simulink library "MyLibTwoSwitchConfig"  (R2024a)
settings: Solver=VariableStepAuto  StartTime=0.0  StopTime=10.0  RelTol=1e-3
values from neighbouring files (symbols this model uses):
  cnt_min = 10    [TX_PM_MODEL_Setup.m]
  cnt_n_bits = 9    [TX_PM_MODEL_Setup.m]
  fH = 2*pi * (fin) / (2*pi - pi/2/N_PHASE_CYCLES)    (= 1066666.66667)    [TX_PM_MODEL_Setup.m]
  fin = 1e6    (= 1000000)    [TX_PM_MODEL_Setup.m]
  fL = 2*pi * (fin) / (2*pi + pi/2/N_PHASE_CYCLES)    (= 941176.470588)    [TX_PM_MODEL_Setup.m]
  R = 0.2    [TX_PM_MODEL_Setup.m]
  tcmp = 5    [TX_PM_MODEL_Setup.m]
  VDD = 5    [Oscillator_Setup.m]    (also in TX_PM_MODEL_Setup.m = 10)
libraries: fl_lib x26, nesl_utility x16, ee_lib x2
settings Model: Creator=ciano  LastModifiedBy=ciano

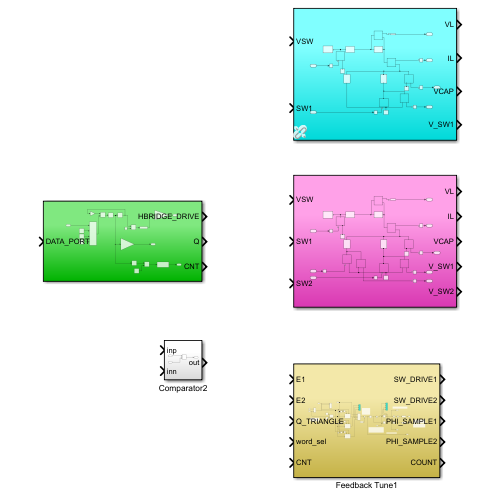
[thumbnail: Simulink's stored preview of the top-level diagram]
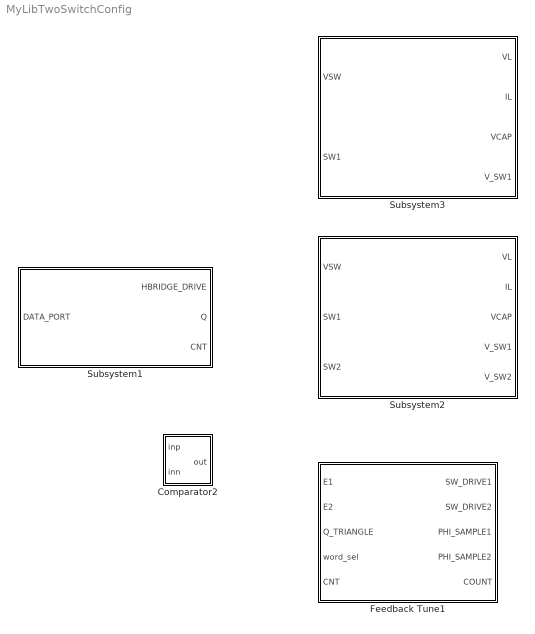
== system MyLibTwoSwitchConfig ==
  Comparator2 : Subsystem
  Feedback Tune1 : Subsystem
  Subsystem1 : Subsystem
  Subsystem2 : Subsystem
  Subsystem3 : Subsystem  AncestorBlock=MyLibTwoSwitchConfig/Subsystem2

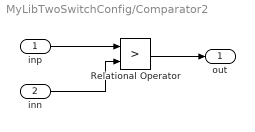
== system MyLibTwoSwitchConfig/Comparator2 ==
  inp : Inport
  inn : Inport  Port=2
  Relational Operator : RelationalOperator  Operator=>  OutDataTypeStr=boolean  RndMeth=Simplest  InputSameDT=off
  out : Outport
  wires:
  inp/1 -> Relational Operator/1
  Relational Operator/1 -> out/1
  inn/1 -> Relational Operator/2

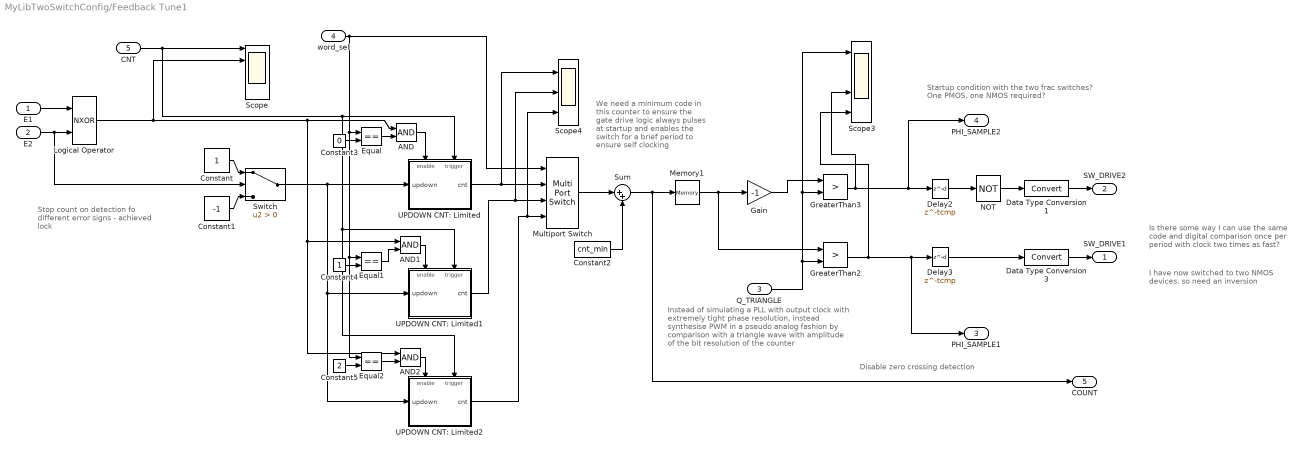
== system MyLibTwoSwitchConfig/Feedback Tune1 ==
  note: Is there some way I can use the same code and digital comparison once per period with clock two times as fast?
  note: We need a minimum code in this counter to ensure the gate drive logic always pulses at startup and enables the switch for a brief period to ensure self clocking
  note: Disable zero crossing detection
  note: Instead of simulating a PLL with output clock with extremely tight phase resolution, instead synthesise PWM in a pseudo analog fashion by comparison with a triangle wave with amplitude of the bit resolution of the counter
  note: Stop count on detection fo different error signs - achieved lock
  note: Startup condition with the two frac switches?
      | One PMOS, one NMOS required?
  note: I have now switched to two NMOS devices. so need an inversion
  E1 : Inport
  E2 : Inport  Port=2
  Q_TRIANGLE : Inport  Port=3
  word_sel : Inport  Port=4
  CNT : Inport  Port=5
  AND : Logic  IconShape=distinctive  AllPortsSameDT=off  OutDataTypeStr=boolean
  AND1 : Logic  IconShape=distinctive  AllPortsSameDT=off  OutDataTypeStr=boolean
  AND2 : Logic  IconShape=distinctive  AllPortsSameDT=off  OutDataTypeStr=boolean
  Constant : Constant
  Constant1 : Constant  Value=-1
  Constant2 : Constant  Value=cnt_min
  Constant3 : Constant  Value=0
  Constant4 : Constant
  Constant5 : Constant  Value=2
  Data Type Conversion1 : DataTypeConversion  SaturateOnIntegerOverflow=off  RndMeth=Floor
  Data Type Conversion3 : DataTypeConversion  SaturateOnIntegerOverflow=off  RndMeth=Floor
  Delay2 : Delay  DelayLength=tcmp  SampleTime=1e-9
  Delay3 : Delay  DelayLength=tcmp  SampleTime=1e-9
  Equal : RelationalOperator  Operator===  OutDataTypeStr=boolean  RndMeth=Simplest  InputSameDT=off
  Equal1 : RelationalOperator  Operator===  OutDataTypeStr=boolean  RndMeth=Simplest  InputSameDT=off
  Equal2 : RelationalOperator  Operator===  OutDataTypeStr=boolean  RndMeth=Simplest  InputSameDT=off
  Gain : Gain  Gain=-1
  GreaterThan2 : RelationalOperator  Operator=>  OutDataTypeStr=boolean  ZeroCross=off  RndMeth=Simplest  InputSameDT=off
  GreaterThan3 : RelationalOperator  Operator=>  OutDataTypeStr=boolean  ZeroCross=off  RndMeth=Simplest  InputSameDT=off
  Logical Operator : Logic  Operator=NXOR  AllPortsSameDT=off  OutDataTypeStr=boolean
  Memory1 : Memory
  Multiport Switch : MultiPortSwitch  DataPortOrder=Zero-based contiguous  zeroidx=on  SaturateOnIntegerOverflow=off  InputSameDT=off
  NOT : Logic  Operator=NOT  IconShape=distinctive  AllPortsSameDT=off  OutDataTypeStr=boolean
  Scope : Scope  NumInputPorts=5
  Scope3 : Scope  NumInputPorts=4
  Scope4 : Scope  NumInputPorts=3
  Sum : Sum  Inputs=|++
  Switch : Switch  Criteria=u2 > Threshold  ZeroCross=off  SaturateOnIntegerOverflow=off  InputSameDT=off
  UPDOWN CNT: Limited : Subsystem
  UPDOWN CNT: Limited1 : Subsystem
  UPDOWN CNT: Limited2 : Subsystem
  SW_DRIVE1 : Outport
  SW_DRIVE2 : Outport  Port=2
  PHI_SAMPLE1 : Outport  Port=3
  PHI_SAMPLE2 : Outport  Port=4
  COUNT : Outport  Port=5
  wires:
  NOT/1 -> Data Type Conversion1/1
  Gain/1 -> GreaterThan3/1
  GreaterThan3/1 -> Scope3/3, Delay2/1, PHI_SAMPLE2/1
  Delay2/1 -> NOT/1
  E1/1 -> Logical Operator/1
  Equal2/1 -> AND2/2
  AND2/1 -> UPDOWN CNT: Limited2/Enable
  Equal1/1 -> AND1/2
  AND1/1 -> UPDOWN CNT: Limited1/Enable
  Equal/1 -> AND/2
  AND/1 -> UPDOWN CNT: Limited/Enable
  Logical Operator/1 -> Scope/2, AND1/1, AND2/1, AND/1
  E2/1 -> Logical Operator/2, Switch/2
  Constant5/1 -> Equal2/2
  Constant4/1 -> Equal1/2
  Constant3/1 -> Equal/2
  UPDOWN CNT: Limited2/1(cnt) -> Multiport Switch/4, Scope4/3
  UPDOWN CNT: Limited1/1(cnt) -> Multiport Switch/3, Scope4/2
  CNT/1 -> Scope/1, UPDOWN CNT: Limited1/Trigger, UPDOWN CNT: Limited2/Trigger, UPDOWN CNT: Limited/Trigger
  Sum/1 -> Memory1/1, COUNT/1
  Multiport Switch/1 -> Sum/1
  Constant2/1 -> Sum/2
  word_sel/1 -> Multiport Switch/1, Equal/1, Equal1/1, Equal2/1
  Q_TRIANGLE/1 -> GreaterThan2/2, Scope3/1, GreaterThan3/2
  GreaterThan2/1 -> Scope3/4, Delay3/1, PHI_SAMPLE1/1
  Delay3/1 -> Data Type Conversion3/1
  Data Type Conversion1/1 -> SW_DRIVE2/1
  Data Type Conversion3/1 -> SW_DRIVE1/1
  Constant1/1 -> Switch/3
  Constant/1 -> Switch/1
  Switch/1 -> UPDOWN CNT: Limited1/1(updown), UPDOWN CNT: Limited2/1(updown), UPDOWN CNT: Limited/1(updown)
  UPDOWN CNT: Limited/1(cnt) -> Multiport Switch/2, Scope4/1
  Memory1/1 -> GreaterThan2/1, Gain/1

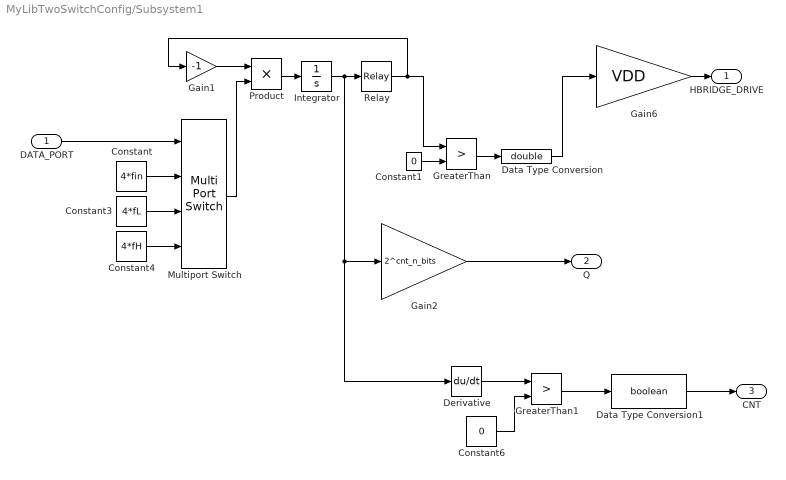
== system MyLibTwoSwitchConfig/Subsystem1 ==
  DATA_PORT : Inport
  Constant : Constant  Value=4*fin
  Constant1 : Constant  Value=0
  Constant3 : Constant  Value=4*fL
  Constant4 : Constant  Value=4*fH
  Constant6 : Constant  Value=0
  Data Type Conversion : DataTypeConversion  OutDataTypeStr=double  SaturateOnIntegerOverflow=off  RndMeth=Floor
  Data Type Conversion1 : DataTypeConversion  OutDataTypeStr=boolean  SaturateOnIntegerOverflow=off  RndMeth=Floor
  Derivative : Derivative
  Gain1 : Gain  Gain=-1
  Gain2 : Gain  Gain=2^cnt_n_bits
  Gain6 : Gain  Gain=VDD
  GreaterThan : RelationalOperator  Operator=>  OutDataTypeStr=boolean  RndMeth=Simplest  InputSameDT=off
  GreaterThan1 : RelationalOperator  Operator=>  OutDataTypeStr=boolean  ZeroCross=off  RndMeth=Simplest  InputSameDT=off
  Integrator : Integrator
  Multiport Switch : MultiPortSwitch  DataPortOrder=Zero-based contiguous  zeroidx=on  SaturateOnIntegerOverflow=off  InputSameDT=off
  Product : Product
  Relay : Relay  OnSwitchValue=1  OffSwitchValue=-1  OffOutputValue=-1
  HBRIDGE_DRIVE : Outport
  Q : Outport  Port=2
  CNT : Outport  Port=3
  wires:
  Gain6/1 -> HBRIDGE_DRIVE/1
  Constant1/1 -> GreaterThan/2
  GreaterThan/1 -> Data Type Conversion/1
  Data Type Conversion/1 -> Gain6/1
  Relay/1 -> Gain1/1, GreaterThan/1
  DATA_PORT/1 -> Multiport Switch/1
  Gain2/1 -> Q/1
  Product/1 -> Integrator/1
  Constant3/1 -> Multiport Switch/3
  Integrator/1 -> Relay/1, Derivative/1, Gain2/1
  Constant4/1 -> Multiport Switch/4
  Constant/1 -> Multiport Switch/2
  Multiport Switch/1 -> Product/2
  Gain1/1 -> Product/1
  Data Type Conversion1/1 -> CNT/1
  Constant6/1 -> GreaterThan1/2
  Derivative/1 -> GreaterThan1/1
  GreaterThan1/1 -> Data Type Conversion1/1

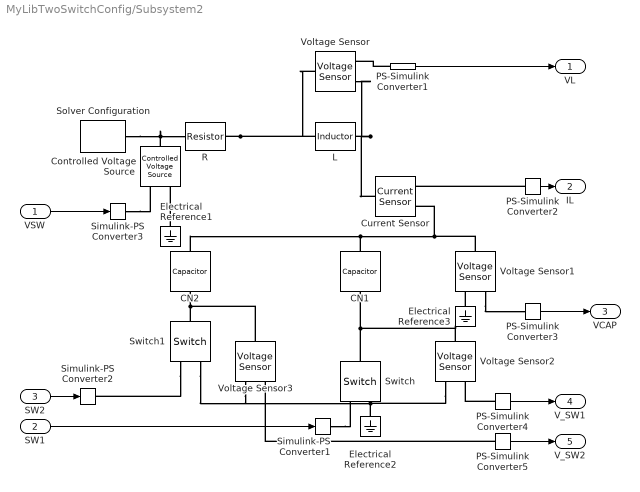
== system MyLibTwoSwitchConfig/Subsystem2 ==
  VSW : Inport
  SW1 : Inport  Port=2
  SW2 : Inport  Port=3
  CN1 : fl_lib/Electrical/Electrical Elements/Capacitor  c=3e-9 F  r=1e-6 Ohm  g=0 1/Ohm  i_specify=off  i_priority=None  i=0 A  i_nominal_specify=off  i_nominal_value=1  i_nominal_unit=A  v_specify=off  v_priority=None  v=0 V  v_nominal_specify=off  v_nominal_value=1  v_nominal_unit=V  vc_specify=off  vc_priority=High  vc=0 V  vc_nominal_specify=off  vc_nominal_value=1  vc_nominal_unit=V
  CN2 : fl_lib/Electrical/Electrical Elements/Capacitor  c=3e-9 F  r=1e-6 Ohm  g=0 1/Ohm  i_specify=off  i_priority=None  i=0 A  i_nominal_specify=off  i_nominal_value=1  i_nominal_unit=A  v_specify=off  v_priority=None  v=0 V  v_nominal_specify=off  v_nominal_value=1  v_nominal_unit=V  vc_specify=off  vc_priority=High  vc=0 V  vc_nominal_specify=off  vc_nominal_value=1  vc_nominal_unit=V
  Controlled Voltage Source : fl_lib/Electrical/Electrical Sources/Controlled Voltage Source
  Current Sensor : fl_lib/Electrical/Electrical Sensors/Current Sensor
  Electrical Reference1 : fl_lib/Electrical/Electrical Elements/Electrical Reference
  Electrical Reference2 : fl_lib/Electrical/Electrical Elements/Electrical Reference
  Electrical Reference3 : fl_lib/Electrical/Electrical Elements/Electrical Reference
  L : ee_lib/Passive/Inductor  l=L H  enable_L_tol=ee.enum.toleranceApplication.none  L_tol=20  tol_distribution=ee.enum.toleranceDistribution.uniform  nSigma=4  r=0 Ohm  g=1e-9 1/Ohm  enable_operating_limits=ee.enum.enable.no  operating_limit_action=ee.enum.passive.reportOpLim.warn  max_working_current=1 A  power_rating=1 W  enable_faults=ee.enum.enable.no  fault_action=simscape.enum.assert.action.none  lambdaPercent=50  k_faulted=0.9999  turnsShort=ee.enum.passive.inductor.turnsShortOption.no  openCct=ee.enum.enable.no  groundShort=ee.enum.passive.inductor.groundShortOption.no  groundShortG=0 1/Ohm  tau_fault=1e-3 s  fault_trigger=ee.enum.faults.faultTrigger.temporal  t_fault=1 s  max_permissible_voltage=100 V  n_fail_on_voltage=1  max_permissible_current=1 A  t_fail_on_current=1 s  i_L_specify=off  i_L_priority=High  i_L=0 A  i_L_nominal_specify=off  i_L_nominal_value=1  i_L_nominal_unit=A  faulted_specify=off  faulted_priority=None  faulted=0
  PS-Simulink Converter{1..5} (5 alike) : nesl_utility/PS-Simulink Converter  PhysicalDomain=network_engine_domain  SubClassName=ps_output  LeftPortType=input  RightPortType=output  PseudoPeriodic=off  Frequencies=[]  VectorFormat=inherit  Unit=inherit  AffineConversion=off
  R : fl_lib/Electrical/Electrical Elements/Resistor  R=R Ohm  i_specify=off  i_priority=None  i=0 A  i_nominal_specify=off  i_nominal_value=1  i_nominal_unit=A  v_specify=off  v_priority=None  v=0 V  v_nominal_specify=off  v_nominal_value=1  v_nominal_unit=V
  Simulink-PS Converter1 : nesl_utility/Simulink-PS Converter  PhysicalDomain=network_engine_domain  SubClassName=ps_input  LeftPortType=input  RightPortType=output  PseudoPeriodic=off  Frequencies=[]  NoiseDistribution=none  NoiseParameters=[]  Unit=1  AffineConversion=off  FilteringAndDerivatives=provide  SimscapeFilterOrder=1  InputFilterTimeConstant=0.001  UdotUserProvided=0
  Simulink-PS Converter2 : nesl_utility/Simulink-PS Converter  PhysicalDomain=network_engine_domain  SubClassName=ps_input  LeftPortType=input  RightPortType=output  PseudoPeriodic=off  Frequencies=[]  NoiseDistribution=none  NoiseParameters=[]  Unit=1  AffineConversion=off  FilteringAndDerivatives=provide  SimscapeFilterOrder=1  InputFilterTimeConstant=0.001  UdotUserProvided=0
  Simulink-PS Converter3 : nesl_utility/Simulink-PS Converter  PhysicalDomain=network_engine_domain  SubClassName=ps_input  LeftPortType=input  RightPortType=output  PseudoPeriodic=off  Frequencies=[]  NoiseDistribution=none  NoiseParameters=[]  Unit=1  AffineConversion=off  FilteringAndDerivatives=provide  SimscapeFilterOrder=1  InputFilterTimeConstant=0.001  UdotUserProvided=0
  Solver Configuration : nesl_utility/Solver Configuration  PhysicalDomain=network_engine_domain  SubClassName=solver  LeftPortType=input  RightPortType=generic  Tones=[]  Harmonics=[]  SimulateNoise=off  Profile=off  UseLocalSampling=off  EnableSwitchedLinearOptims=on  FrequencyDomain=off  UseCCode=off  RelTol=0.001  AbsTol=0.001  MinStep=1e-09  ToWorkspace=off  RevertToSquareIcSolve=off  NumHomotopyIterations=100  PhasorMode=off  PhasorModeNumHarmonics=1  ConsistencySolver=NEWTON_XTOL_AFTER_FTOL  IndexReductionMethod=DerivativeReplacement  DoDC=off  ResidualTolerance=1e-09  ConsistencyTolSource=GLOBAL  ConsistencyAbsTol=0.001  ConsistencyRelTol=0.001  ConsistencyTolFactor=0.001  UseLocalSolver=off  LocalSolverChoice=NE_BACKWARD_EULER_ADVANCER  ResolveIndetEquations=on  FunctionEvalNumThread=1  LocalSolverSampleTime=0.001  DoFixedCost=off  MaxNonlinIter=3  MaxModeIter=2  ComputeImpulses=off  ImpulseIterations=2  LinearAlgebra=auto  LinearAlgebraNumThread=0  EquationFormulation=NE_TIME_EF  DelaysMemoryBudget=1024  AutomaticFiltering=on  FilteringTimeConstant=0.001  PartitionStorageMethod=AS_NEEDED  PartitionMemoryBudget=1024  PartitionMethod=ROBUST  MultibodyUseLocalSolver=off  MultibodyLocalSolverChoice=ODE1  MultibodyLocalSolverSampleTime=0.001
  Switch : fl_lib/Electrical/Electrical Elements/Switch  R_closed=0.1 Ohm  G_open=1e-8 1/Ohm  Threshold=0.5  i_specify=off  i_priority=None  i=0 A  i_nominal_specify=off  i_nominal_value=1  i_nominal_unit=A  v_specify=off  v_priority=None  v=0 V  v_nominal_specify=off  v_nominal_value=1  v_nominal_unit=V
  Switch1 : fl_lib/Electrical/Electrical Elements/Switch  R_closed=0.01 Ohm  G_open=1e-8 1/Ohm  Threshold=0.5  i_specify=off  i_priority=None  i=0 A  i_nominal_specify=off  i_nominal_value=1  i_nominal_unit=A  v_specify=off  v_priority=None  v=0 V  v_nominal_specify=off  v_nominal_value=1  v_nominal_unit=V
  Voltage Sensor{,1..3} (4 alike) : fl_lib/Electrical/Electrical Sensors/Voltage Sensor
  VL : Outport
  IL : Outport  Port=2
  VCAP : Outport  Port=3
  V_SW1 : Outport  Port=4
  V_SW2 : Outport  Port=5
  wires:
  PS-Simulink Converter1/1 -> VL/1
  VSW/1 -> Simulink-PS Converter3/1
  PS-Simulink Converter4/1 -> V_SW1/1
  PS-Simulink Converter2/1 -> IL/1
  SW1/1 -> Simulink-PS Converter1/1
  PS-Simulink Converter3/1 -> VCAP/1
  SW2/1 -> Simulink-PS Converter2/1
  PS-Simulink Converter5/1 -> V_SW2/1
  connections:
  Solver Configuration/RConn1 -- R/LConn1 -- Controlled Voltage Source/LConn1
  R/RConn1 -- Voltage Sensor/LConn1 -- L/LConn1
  PS-Simulink Converter4/LConn1 -- Voltage Sensor2/RConn1
  Simulink-PS Converter1/RConn1 -- Switch/RConn1
  Voltage Sensor2/RConn2 -- Voltage Sensor3/RConn2 -- Switch1/RConn2 -- Switch/RConn2 -- Electrical Reference2/LConn1
  PS-Simulink Converter1/LConn1 -- Voltage Sensor/RConn1
  PS-Simulink Converter2/LConn1 -- Current Sensor/RConn1
  CN2/LConn1 -- Current Sensor/RConn2 -- Voltage Sensor1/LConn1 -- CN1/LConn1
  Simulink-PS Converter3/RConn1 -- Controlled Voltage Source/RConn1
  Switch/LConn1 -- Voltage Sensor2/LConn1 -- CN1/RConn1
  Electrical Reference3/LConn1 -- Voltage Sensor1/RConn2
  Voltage Sensor1/RConn1 -- PS-Simulink Converter3/LConn1
  Electrical Reference1/LConn1 -- Controlled Voltage Source/RConn2
  L/RConn1 -- Voltage Sensor/RConn2 -- Current Sensor/LConn1
  Switch1/LConn1 -- Voltage Sensor3/LConn1 -- CN2/RConn1
  Switch1/RConn1 -- Simulink-PS Converter2/RConn1
  PS-Simulink Converter5/LConn1 -- Voltage Sensor3/RConn1

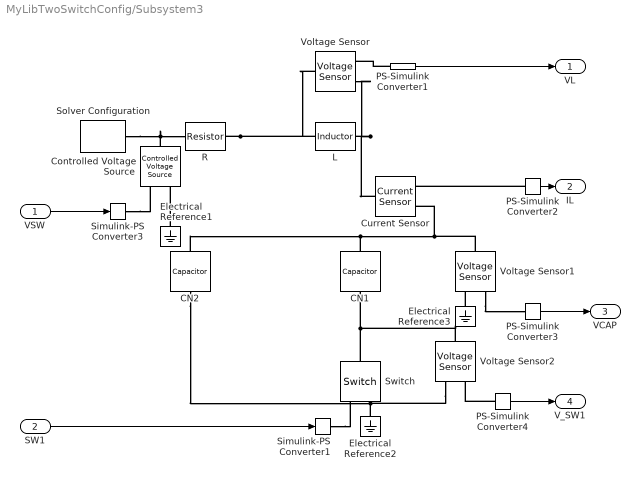
== system MyLibTwoSwitchConfig/Subsystem3 ==
  VSW : Inport
  SW1 : Inport  Port=2
  CN1 : fl_lib/Electrical/Electrical Elements/Capacitor  c=3e-9 F  r=1e-6 Ohm  g=0 1/Ohm  i_specify=off  i_priority=None  i=0 A  i_nominal_specify=off  i_nominal_value=1  i_nominal_unit=A  v_specify=off  v_priority=None  v=0 V  v_nominal_specify=off  v_nominal_value=1  v_nominal_unit=V  vc_specify=off  vc_priority=High  vc=0 V  vc_nominal_specify=off  vc_nominal_value=1  vc_nominal_unit=V
  CN2 : fl_lib/Electrical/Electrical Elements/Capacitor  c=3e-9 F  r=1e-6 Ohm  g=0 1/Ohm  i_specify=off  i_priority=None  i=0 A  i_nominal_specify=off  i_nominal_value=1  i_nominal_unit=A  v_specify=off  v_priority=None  v=0 V  v_nominal_specify=off  v_nominal_value=1  v_nominal_unit=V  vc_specify=off  vc_priority=High  vc=0 V  vc_nominal_specify=off  vc_nominal_value=1  vc_nominal_unit=V
  Controlled Voltage Source : fl_lib/Electrical/Electrical Sources/Controlled Voltage Source
  Current Sensor : fl_lib/Electrical/Electrical Sensors/Current Sensor
  Electrical Reference1 : fl_lib/Electrical/Electrical Elements/Electrical Reference
  Electrical Reference2 : fl_lib/Electrical/Electrical Elements/Electrical Reference
  Electrical Reference3 : fl_lib/Electrical/Electrical Elements/Electrical Reference
  L : ee_lib/Passive/Inductor  l=L H  enable_L_tol=ee.enum.toleranceApplication.none  L_tol=20  tol_distribution=ee.enum.toleranceDistribution.uniform  nSigma=4  r=0 Ohm  g=1e-9 1/Ohm  enable_operating_limits=ee.enum.enable.no  operating_limit_action=ee.enum.passive.reportOpLim.warn  max_working_current=1 A  power_rating=1 W  enable_faults=ee.enum.enable.no  fault_action=simscape.enum.assert.action.none  lambdaPercent=50  k_faulted=0.9999  turnsShort=ee.enum.passive.inductor.turnsShortOption.no  openCct=ee.enum.enable.no  groundShort=ee.enum.passive.inductor.groundShortOption.no  groundShortG=0 1/Ohm  tau_fault=1e-3 s  fault_trigger=ee.enum.faults.faultTrigger.temporal  t_fault=1 s  max_permissible_voltage=100 V  n_fail_on_voltage=1  max_permissible_current=1 A  t_fail_on_current=1 s  i_L_specify=off  i_L_priority=High  i_L=0 A  i_L_nominal_specify=off  i_L_nominal_value=1  i_L_nominal_unit=A  faulted_specify=off  faulted_priority=None  faulted=0
  PS-Simulink Converter{1..4} (4 alike) : nesl_utility/PS-Simulink Converter  PhysicalDomain=network_engine_domain  SubClassName=ps_output  LeftPortType=input  RightPortType=output  PseudoPeriodic=off  Frequencies=[]  VectorFormat=inherit  Unit=inherit  AffineConversion=off
  R : fl_lib/Electrical/Electrical Elements/Resistor  R=R Ohm  i_specify=off  i_priority=None  i=0 A  i_nominal_specify=off  i_nominal_value=1  i_nominal_unit=A  v_specify=off  v_priority=None  v=0 V  v_nominal_specify=off  v_nominal_value=1  v_nominal_unit=V
  Simulink-PS Converter1 : nesl_utility/Simulink-PS Converter  PhysicalDomain=network_engine_domain  SubClassName=ps_input  LeftPortType=input  RightPortType=output  PseudoPeriodic=off  Frequencies=[]  NoiseDistribution=none  NoiseParameters=[]  Unit=1  AffineConversion=off  FilteringAndDerivatives=provide  SimscapeFilterOrder=1  InputFilterTimeConstant=0.001  UdotUserProvided=0
  Simulink-PS Converter3 : nesl_utility/Simulink-PS Converter  PhysicalDomain=network_engine_domain  SubClassName=ps_input  LeftPortType=input  RightPortType=output  PseudoPeriodic=off  Frequencies=[]  NoiseDistribution=none  NoiseParameters=[]  Unit=1  AffineConversion=off  FilteringAndDerivatives=provide  SimscapeFilterOrder=1  InputFilterTimeConstant=0.001  UdotUserProvided=0
  Solver Configuration : nesl_utility/Solver Configuration  PhysicalDomain=network_engine_domain  SubClassName=solver  LeftPortType=input  RightPortType=generic  Tones=[]  Harmonics=[]  SimulateNoise=off  Profile=off  UseLocalSampling=off  EnableSwitchedLinearOptims=on  FrequencyDomain=off  UseCCode=off  RelTol=0.001  AbsTol=0.001  MinStep=1e-09  ToWorkspace=off  RevertToSquareIcSolve=off  NumHomotopyIterations=100  PhasorMode=off  PhasorModeNumHarmonics=1  ConsistencySolver=NEWTON_XTOL_AFTER_FTOL  IndexReductionMethod=DerivativeReplacement  DoDC=off  ResidualTolerance=1e-09  ConsistencyTolSource=GLOBAL  ConsistencyAbsTol=0.001  ConsistencyRelTol=0.001  ConsistencyTolFactor=0.001  UseLocalSolver=off  LocalSolverChoice=NE_BACKWARD_EULER_ADVANCER  ResolveIndetEquations=on  FunctionEvalNumThread=1  LocalSolverSampleTime=0.001  DoFixedCost=off  MaxNonlinIter=3  MaxModeIter=2  ComputeImpulses=off  ImpulseIterations=2  LinearAlgebra=auto  LinearAlgebraNumThread=0  EquationFormulation=NE_TIME_EF  DelaysMemoryBudget=1024  AutomaticFiltering=on  FilteringTimeConstant=0.001  PartitionStorageMethod=AS_NEEDED  PartitionMemoryBudget=1024  PartitionMethod=ROBUST  MultibodyUseLocalSolver=off  MultibodyLocalSolverChoice=ODE1  MultibodyLocalSolverSampleTime=0.001
  Switch : fl_lib/Electrical/Electrical Elements/Switch  R_closed=0.1 Ohm  G_open=1e-8 1/Ohm  Threshold=0.5  i_specify=off  i_priority=None  i=0 A  i_nominal_specify=off  i_nominal_value=1  i_nominal_unit=A  v_specify=off  v_priority=None  v=0 V  v_nominal_specify=off  v_nominal_value=1  v_nominal_unit=V
  Voltage Sensor : fl_lib/Electrical/Electrical Sensors/Voltage Sensor
  Voltage Sensor1 : fl_lib/Electrical/Electrical Sensors/Voltage Sensor
  Voltage Sensor2 : fl_lib/Electrical/Electrical Sensors/Voltage Sensor
  VL : Outport
  IL : Outport  Port=2
  VCAP : Outport  Port=3
  V_SW1 : Outport  Port=4
  wires:
  PS-Simulink Converter1/1 -> VL/1
  VSW/1 -> Simulink-PS Converter3/1
  PS-Simulink Converter4/1 -> V_SW1/1
  PS-Simulink Converter2/1 -> IL/1
  SW1/1 -> Simulink-PS Converter1/1
  PS-Simulink Converter3/1 -> VCAP/1
  connections:
  Solver Configuration/RConn1 -- R/LConn1 -- Controlled Voltage Source/LConn1
  R/RConn1 -- Voltage Sensor/LConn1 -- L/LConn1
  PS-Simulink Converter4/LConn1 -- Voltage Sensor2/RConn1
  Simulink-PS Converter1/RConn1 -- Switch/RConn1
  PS-Simulink Converter1/LConn1 -- Voltage Sensor/RConn1
  PS-Simulink Converter2/LConn1 -- Current Sensor/RConn1
  CN2/LConn1 -- Current Sensor/RConn2 -- Voltage Sensor1/LConn1 -- CN1/LConn1
  Simulink-PS Converter3/RConn1 -- Controlled Voltage Source/RConn1
  Switch/LConn1 -- Voltage Sensor2/LConn1 -- CN1/RConn1
  Electrical Reference3/LConn1 -- Voltage Sensor1/RConn2
  Voltage Sensor1/RConn1 -- PS-Simulink Converter3/LConn1
  Electrical Reference1/LConn1 -- Controlled Voltage Source/RConn2
  L/RConn1 -- Voltage Sensor/RConn2 -- Current Sensor/LConn1
  Voltage Sensor2/RConn2 -- CN2/RConn1 -- Switch/RConn2 -- Electrical Reference2/LConn1

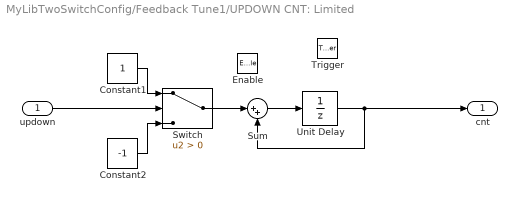
== system MyLibTwoSwitchConfig/Feedback Tune1/UPDOWN CNT: Limited ==
  updown : Inport
  Enable : EnablePort
  Trigger : TriggerPort  TriggerType=either  VariantControl=(inherit)  PortDimensions=1
  Constant1 : Constant
  Constant2 : Constant  Value=-1
  Sum : Sum  Inputs=|++
  Switch : Switch  Criteria=u2 > Threshold  SaturateOnIntegerOverflow=off  InputSameDT=off
  Unit Delay : UnitDelay  SampleTime=-1  HasFrameUpgradeWarning=on
  cnt : Outport
  wires:
  Unit Delay/1 -> Sum/2, cnt/1
  Constant1/1 -> Switch/1
  updown/1 -> Switch/2
  Sum/1 -> Unit Delay/1
  Constant2/1 -> Switch/3
  Switch/1 -> Sum/1

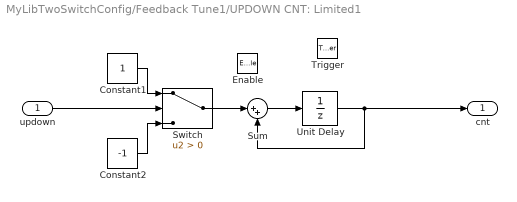
== system MyLibTwoSwitchConfig/Feedback Tune1/UPDOWN CNT: Limited1 ==
  updown : Inport
  Enable : EnablePort
  Trigger : TriggerPort  TriggerType=either  VariantControl=(inherit)  PortDimensions=1
  Constant1 : Constant
  Constant2 : Constant  Value=-1
  Sum : Sum  Inputs=|++
  Switch : Switch  Criteria=u2 > Threshold  SaturateOnIntegerOverflow=off  InputSameDT=off
  Unit Delay : UnitDelay  SampleTime=-1  HasFrameUpgradeWarning=on
  cnt : Outport
  wires:
  Unit Delay/1 -> Sum/2, cnt/1
  Constant1/1 -> Switch/1
  updown/1 -> Switch/2
  Sum/1 -> Unit Delay/1
  Constant2/1 -> Switch/3
  Switch/1 -> Sum/1

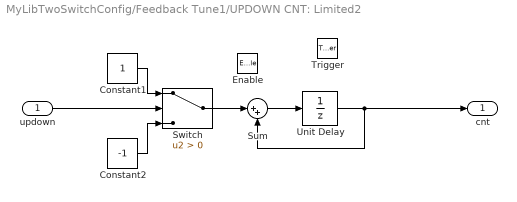
== system MyLibTwoSwitchConfig/Feedback Tune1/UPDOWN CNT: Limited2 ==
  updown : Inport
  Enable : EnablePort
  Trigger : TriggerPort  TriggerType=either  VariantControl=(inherit)  PortDimensions=1
  Constant1 : Constant
  Constant2 : Constant  Value=-1
  Sum : Sum  Inputs=|++
  Switch : Switch  Criteria=u2 > Threshold  SaturateOnIntegerOverflow=off  InputSameDT=off
  Unit Delay : UnitDelay  SampleTime=-1  HasFrameUpgradeWarning=on
  cnt : Outport
  wires:
  Unit Delay/1 -> Sum/2, cnt/1
  Constant1/1 -> Switch/1
  updown/1 -> Switch/2
  Sum/1 -> Unit Delay/1
  Constant2/1 -> Switch/3
  Switch/1 -> Sum/1
